simulink model "Ex9_11model"  (R2013a)
settings: Solver=ode3  StartTime=0.0  StopTime=2  FixedStep=.001  RelTol=1e-3
settings Model: Creator=JLS  LastModifiedBy=John
settings DataIOCC: SignalLoggingSaveFormat=ModelDataLogs
settings OptimizationCC: ExpressionDepthLimit=2147483647
settings DebuggingCC: FcnCallInpInsideContextMsg=UseLocalSettings
settings GRTTargetCC: CombineOutputUpdateFcns=off  GRTInterface=on

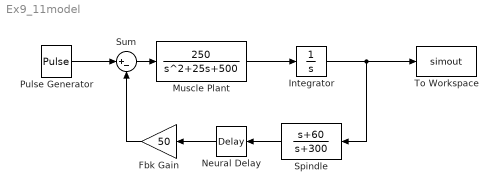
== system Ex9_11model ==
  Fbk Gain : Gain  Gain=50
  Integrator : Integrator
  Muscle Plant : TransferFcn  Numerator=250  Denominator=[1 25 500]
  Neural Delay : TransportDelay  DelayTime=.03
  Pulse Generator : DiscretePulseGenerator  PulseType=Time based  Period=3
  Spindle : TransferFcn  Numerator=[1 60]  Denominator=[1 300]
  Sum : Sum  Inputs=|+-
  To Workspace : ToWorkspace  VariableName=simout  SampleTime=-1
  wires:
  Sum/1 -> Muscle Plant/1
  Muscle Plant/1 -> Integrator/1
  Integrator/1 -> To Workspace/1, Spindle/1
  Fbk Gain/1 -> Sum/2
  Pulse Generator/1 -> Sum/1
  Neural Delay/1 -> Fbk Gain/1
  Spindle/1 -> Neural Delay/1
